simulink model "simulazione_sistema_non_lineare"  (R2025b)
settings: Solver=VariableStepAuto  StartTime=0.0  StopTime=10.0  RelTol=1e-3
values from neighbouring files (symbols this model uses):
  D = 0    [simulazione_sistema_non_lineare_code.m]    (also in tank_in_cascata_costanti.m; tank_test_disturbo_dominio_tempo.m = 1.5; tank_test_disturbo_uscita.m = 1.5)
  N = 0    [simulazione_sistema_non_lineare_code.m]    (also in tank_test_disturbo_dominio_tempo.m = 0.1; tank_test_disturbo_uscita.m = 0.1)
  U = [0 1]    [simulazione_sistema_non_lineare_code.m]
  ue = (k1/k4)*sqrt(xe(1))    [tank_in_cascata_costanti.m]
  W = 3.5    [animazione_regolatore.m]    (also in simulazione_sistema_lineare_code.m = 1; simulazione_sistema_non_lineare_code.m = 1; tank_test_disturbo_dominio_complesso.m; tank_test_disturbo_dominio_tempo.m)
  xe = [9.45, 4.20]    [tank_in_cascata_costanti.m]
libraries: cstblocks x1
settings Model: Creator=lucia  LastModifiedBy=lucia

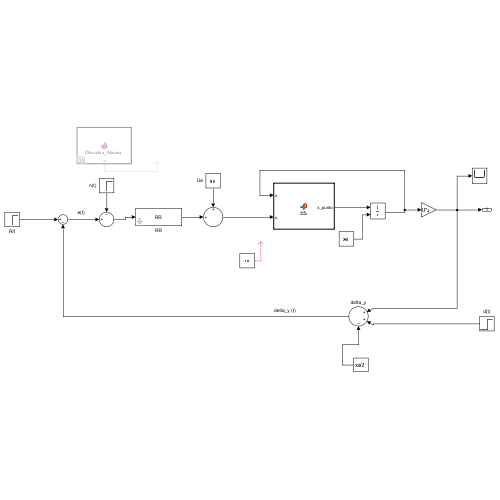
[thumbnail: Simulink's stored preview of the top-level diagram]
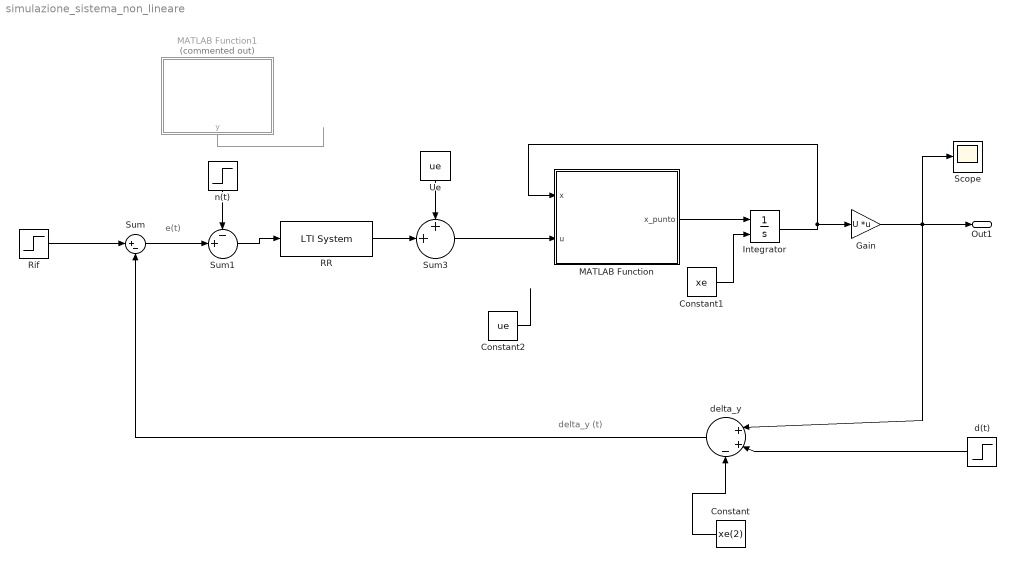
== system simulazione_sistema_non_lineare ==
  note: delta_y (t)
  note: e(t)
  Constant : Constant  Value=xe(2)
  Constant1 : Constant  Value=xe
  Constant2 : Constant  Value=ue
  Gain : Gain  Gain=U  Multiplication=Matrix(K*u)
  Integrator : Integrator  InitialConditionSource=external
  MATLAB Function : MATLAB Function  TreatAsAtomicUnit=on
  MATLAB Function1 : MATLAB Function  Commented=on  TreatAsAtomicUnit=on
  RR : cstblocks/LTI System  sys=RR  IC=[]  PadeOrder=0
  Rif : Step  After=W  SampleTime=0
  Scope : Scope
      settings: ActiveDisplayYMinimum=3.5643480963669694  ActiveDisplayYMaximum=7.3620581654159052
  Sum : Sum  Inputs=|+-
  Sum1 : Sum  Inputs=-+|
  Sum3 : Sum  Inputs=++|
  Ue : Constant  Value=ue
  d(t) : Step  After=D  SampleTime=0
  delta_y : Sum  Inputs=|++-
  n(t) : Step  After=N  SampleTime=0
  Out1 : Outport
  wires:
  MATLAB Function/1(x_punto) -> Integrator/1
  RR/1 -> Sum3/2
  Sum3/1 -> MATLAB Function/2(u)
  Ue/1 -> Sum3/1
  Constant/1 -> delta_y/3
  delta_y/1 -> Sum/2
  Rif/1 -> Sum/1
  Integrator/1 -> Gain/1, MATLAB Function/1(x)
  Sum/1 -> Sum1/2
  Constant1/1 -> Integrator/2
  d(t)/1 -> delta_y/2
  n(t)/1 -> Sum1/1
  Sum1/1 -> RR/1
  Gain/1 -> Out1/1, Scope/1, delta_y/1
  Constant2/1 -> ?
  MATLAB Function1/1(y) -> ?

== matlab function simulazione_sistema_non_lineare/MATLAB Function1 ==
  data: y output
function y = Disturbo_Misura()
N = 1;
omega = 0.4;
phase = 0;
n_t = 0;

for n = 1:4
    omega_n = omega*n;
    phase_n = phase*n;
    n_t = n_t + N*sin(omega_n*t+phase_n); 
end

y = n_t;
end

== matlab function simulazione_sistema_non_lineare/MATLAB Function ==
  data: x input; x_punto output; u input
function x_punto = SS(x,u)
% Costanti del sistema
k1=1;
k2=0.30;
k3=0.45;
k4=0.50;

x_punto = zeros(2,1);

%sistema in forma di stato
x_punto(1) = real(-k1*sqrt(complex(x(1))) + k4*u);
x_punto(2) = real(k2*sqrt(complex(x(1))) - k3*sqrt(complex(x(2))));

end
